simulink model "FinalPIDSensorFusion6DOF"  (R2024b)
settings: Solver=VariableStepAuto  StartTime=0.0  StopTime=5.0  RelTol=1e-3
libraries: aerolibnav x2, shared6dof x1
settings Model: Creator=ARULPAVALAN S A  LastModifiedBy=ARULPAVALAN S A

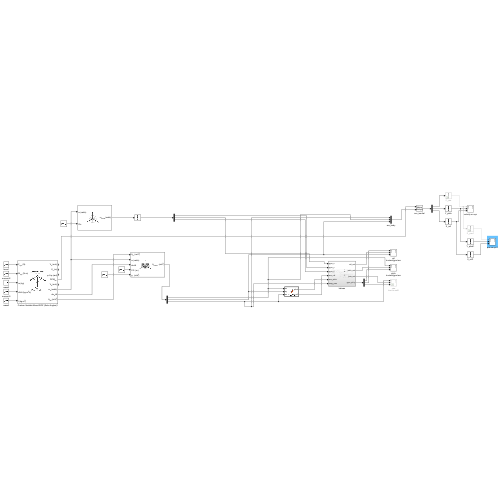
[thumbnail: Simulink's stored preview of the top-level diagram]
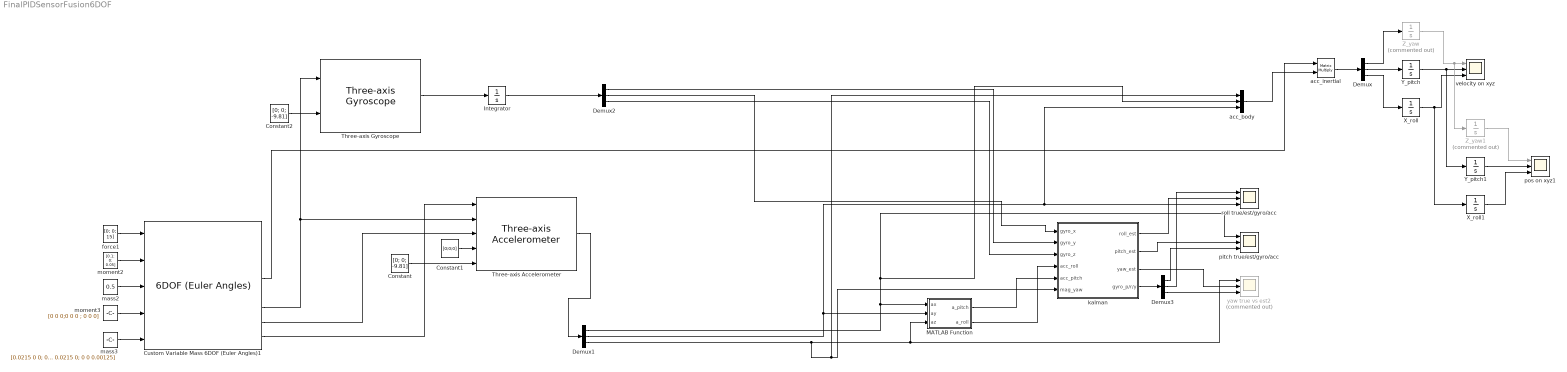
== system FinalPIDSensorFusion6DOF ==
  Constant : Constant  Value=[0; 0; -9.81]
  Constant1 : Constant  Value=[0;0;0]
  Constant2 : Constant  Value=[0; 0; -9.81]
  Custom Variable Mass 6DOF (Euler Angles)1 : shared6dof/6DOF (Euler Angles)  units=Metric (MKS)  mtype=Custom Variable  rep=Euler Angles  xme_0=[0 0 0]  Vm_0=[0 0 0]  eul_0=[0 0 0]  pm_0=[0 0 0]  mass_0=1.0  mass_e=0.5  mass_f=2.0  inertia=eye(3)  inertia_e=eye(3)  inertia_f=2*eye(3)  k_quat=1.0  vre_flag=off  abi_flag=off  aMode=0  xme_statename=''  Vm_statename=''  eul_statename=''  quat_statename=''  pm_statename=''  mass_statename=''
      settings: LibrarySourceBlock=aerolib6dof2/Custom Variable Mass 6DOF (Euler Angles)
  Demux{,1..3} (4 alike) : Demux  Outputs=3
  Integrator : Integrator
  MATLAB Function : MATLAB Function  TreatAsAtomicUnit=on
  Three-axis Accelerometer : aerolibnav/Three-axis Accelerometer  units=Metric (MKS)  acc=[0 0 0]  gtype=on  dtype_a=on  w_a=190  z_a=0.707  a_sf_cc=[1 0 0; 0 1 0; 0 0 1]  a_bias=[0 0 0]  a_Ts=0  a_rand=on  a_seeds=[23093 23094 23095]  a_pow=[0.001 0.001 0.001]  a_sat="[-inf  -inf  -inf  inf inf inf]"
  Three-axis Gyroscope : aerolibnav/Three-axis Gyroscope  dtype_g=on  w_g=190  z_g=0.707  g_sf_cc=[1 0 0; 0 1 0; 0 0 1]  g_bias=[0 0 0]  g_sen=[0 0 0]  g_Ts=0  g_rand=on  g_seeds=[23093 23094 23095]  g_pow=[0.0001 0.0001 0.0001]  g_sat="[-inf  -inf  -inf  inf inf inf]"
  X_roll : Integrator
  X_roll1 : Integrator
  Y_pitch : Integrator
  Y_pitch1 : Integrator
  Z_yaw : Integrator  Commented=on
  Z_yaw1 : Integrator  Commented=on
  acc_body : Mux  Inputs=3
  acc_inertial : Product  Multiplication=Matrix(*)
  force1 : Constant  Value=[0; 0; 15]
  kalman : Subsystem
  mass2 : Constant  Value=0.5
  mass3 : Constant  Value=[0.0215 0 0; 0 0.0215 0; 0 0 0.00125]
  moment2 : Constant  Value=[0.1; 0; 0.05]
  moment3 : Constant  Value=[0 0 0;0 0 0 ; 0 0 0]
  pitch true/est/gyro/acc : Scope  NumInputPorts=3
  pos on xyz1 : Scope  NumInputPorts=3
  roll true/est/gyro/acc : Scope  NumInputPorts=3
  velocity on xyz : Scope  NumInputPorts=3
  yaw true vs est2 : Scope  Commented=on  NumInputPorts=3
  wires:
  Demux2/1 -> kalman/2(gyro_y)
  kalman/2(pitch_est) -> pitch true/est/gyro/acc/2
  Demux1/1 -> pitch true/est/gyro/acc/1, acc_body/2, MATLAB Function/1(ax)
  Demux1/2 -> MATLAB Function/2(ay), acc_body/3, roll true/est/gyro/acc/3
  kalman/3(yaw_est) -> yaw true vs est2/2
  Demux2/3 -> kalman/3(gyro_z)
  Demux1/3 -> MATLAB Function/3(az), yaw true vs est2/1, acc_body/1, kalman/6(mag_yaw)
  acc_body/1 -> acc_inertial/2
  acc_inertial/1 -> Demux/1
  Demux/2 -> Y_pitch/1
  Demux/1 -> Z_yaw/1
  Demux/3 -> X_roll/1
  X_roll/1 -> X_roll1/1, velocity on xyz/3
  Y_pitch/1 -> Y_pitch1/1, velocity on xyz/2
  Y_pitch1/1 -> pos on xyz1/2
  X_roll1/1 -> pos on xyz1/3
  mass3/1 -> Custom Variable Mass 6DOF (Euler Angles)1/5
  moment2/1 -> Custom Variable Mass 6DOF (Euler Angles)1/2
  moment3/1 -> Custom Variable Mass 6DOF (Euler Angles)1/4
  force1/1 -> Custom Variable Mass 6DOF (Euler Angles)1/1
  mass2/1 -> Custom Variable Mass 6DOF (Euler Angles)1/3
  Custom Variable Mass 6DOF (Euler Angles)1/4 -> acc_inertial/1
  Custom Variable Mass 6DOF (Euler Angles)1/8 -> Three-axis Accelerometer/1
  Custom Variable Mass 6DOF (Euler Angles)1/6 -> Three-axis Accelerometer/2, Three-axis Gyroscope/1
  kalman/1(roll_est) -> roll true/est/gyro/acc/2
  kalman/4(gyro_p/r/y) -> Demux3/1
  Demux3/2 -> roll true/est/gyro/acc/1
  Custom Variable Mass 6DOF (Euler Angles)1/7 -> Three-axis Accelerometer/3
  Constant/1 -> Three-axis Accelerometer/5
  Constant1/1 -> Three-axis Accelerometer/4
  Three-axis Accelerometer/1 -> Demux1/1
  Demux3/1 -> pitch true/est/gyro/acc/3
  Demux3/3 -> yaw true vs est2/3
  Constant2/1 -> Three-axis Gyroscope/2
  MATLAB Function/1(a_pitch) -> kalman/5(acc_pitch)
  MATLAB Function/2(a_roll) -> kalman/4(acc_roll)
  Demux2/2 -> kalman/1(gyro_x)
  Integrator/1 -> Demux2/1
  Three-axis Gyroscope/1 -> Integrator/1
  Z_yaw/1 -> Z_yaw1/1, velocity on xyz/1
  Z_yaw1/1 -> pos on xyz1/1

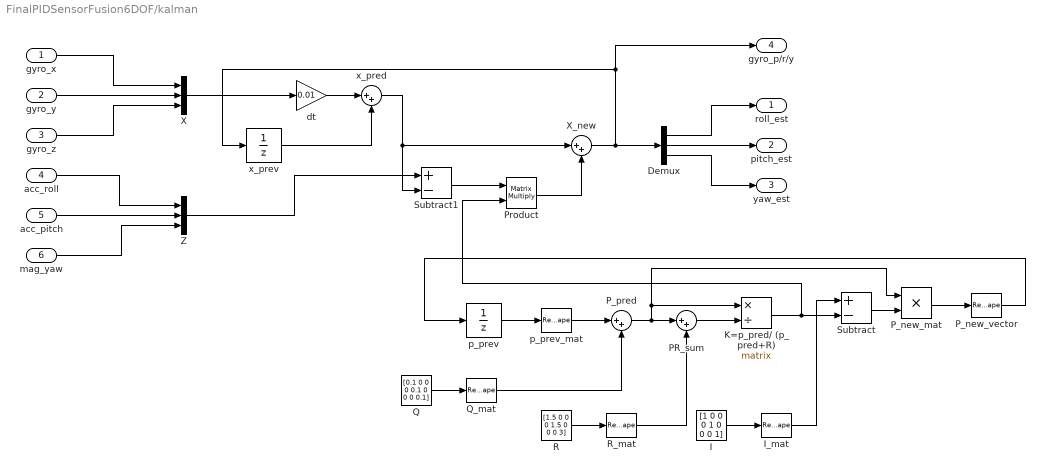
== system FinalPIDSensorFusion6DOF/kalman ==
  gyro_x : Inport
  gyro_y : Inport  Port=2
  gyro_z : Inport  Port=3
  acc_roll : Inport  Port=4
  acc_pitch : Inport  Port=5
  mag_yaw : Inport  Port=6
  Demux : Demux  Outputs=3
  I : Constant  Value=[1 0 0 0 1 0 0 0 1]
  I_mat : Reshape  OutputDimensionality=Customize  OutputDimensions=[3,3]
  K=p_pred/ (p_pred+R) : Product  Inputs=*/  Multiplication=Matrix(*)
  "PR_sum " : Sum  Inputs=|++
  P_new_mat : Product
  P_new_vector : Reshape  OutputDimensionality=Customize  OutputDimensions=[1,9]
  "P_pred " : Sum  Inputs=|++
  Product : Product  Multiplication=Matrix(*)
  Q : Constant  Value=[0.1 0 0 0 0.1 0 0 0 0.1]
  Q_mat : Reshape  OutputDimensionality=Customize  OutputDimensions=[3,3]
  R : Constant  Value=[1.5 0 0 0 1.5 0 0 0 3]
  R_mat : Reshape  OutputDimensionality=Customize  OutputDimensions=[3,3]
  Subtract : Sum  Inputs=+-
  Subtract1 : Sum  Inputs=+-
  X : Mux  Inputs=3
  X_new : Sum  Inputs=|++
  Z : Mux  Inputs=3
  dt : Gain  Gain=0.01
  p_prev : UnitDelay  InitialCondition=[1 0 0 0 1 0 0 0 1]  SampleTime=-1  HasFrameUpgradeWarning=on
  p_prev_mat : Reshape  OutputDimensionality=Customize  OutputDimensions=[3,3]
  "x_pred " : Sum  Inputs=|++
  x_prev : UnitDelay  SampleTime=-1  HasFrameUpgradeWarning=on
  roll_est : Outport
  pitch_est : Outport  Port=2
  yaw_est : Outport  Port=3
  gyro_p/r/y : Outport  Port=4
  wires:
  R_mat/1 -> "PR_sum "/2
  Subtract/1 -> P_new_mat/2
  X_new/1 -> Demux/1, gyro_p/r/y/1, x_prev/1
  "PR_sum "/1 -> K=p_pred/ (p_pred+R)/2
  K=p_pred/ (p_pred+R)/1 -> Product/2, Subtract/2
  "P_pred "/1 -> P_new_mat/1, K=p_pred/ (p_pred+R)/1, "PR_sum "/1
  R/1 -> R_mat/1
  X/1 -> dt/1
  mag_yaw/1 -> Z/3
  "x_pred "/1 -> X_new/1, Subtract1/2
  P_new_mat/1 -> P_new_vector/1
  acc_roll/1 -> Z/1
  Q/1 -> Q_mat/1
  Subtract1/1 -> Product/1
  Demux/1 -> roll_est/1
  Demux/3 -> yaw_est/1
  Q_mat/1 -> "P_pred "/2
  I_mat/1 -> Subtract/1
  gyro_z/1 -> X/3
  p_prev/1 -> p_prev_mat/1
  p_prev_mat/1 -> "P_pred "/1
  Product/1 -> X_new/2
  x_prev/1 -> "x_pred "/2
  dt/1 -> "x_pred "/1
  gyro_x/1 -> X/1
  P_new_vector/1 -> p_prev/1
  Demux/2 -> pitch_est/1
  I/1 -> I_mat/1
  acc_pitch/1 -> Z/2
  gyro_y/1 -> X/2
  Z/1 -> Subtract1/1

== matlab function FinalPIDSensorFusion6DOF/MATLAB Function ==
  data: ax input; a_pitch output; ay input; az input; a_roll output
function [a_pitch, a_roll] = acl_ang(ax, ay, az)

a_roll = atan2d(ay, az);


a_pitch = atan2d(-ax, sqrt(ay^2 + az^2));
end
